simulink model "dynamicANN"  (R2019b)
settings: Solver=VariableStepAuto  StartTime=0.0  StopTime=3  RelTol=1e-3
values from neighbouring files (symbols this model uses):
  a = 87.548e-3    (= 0.087548)    [main.m]
  b = 132.452e-3    (= 0.132452)    [main.m]
  d = 22.452e-3    (= 0.022452)    [main.m]
  delta = 4e-6    (= 4e-06)    [main.m]
  F1 = mass*g-F2    (= 23.4474357109)    [main.m]
  F2 = a*mass*g/(a+b)    (= 15.4982642891)    [main.m]
  g = 9.81    [main.m]
  h0 = 75e-6    (= 7.5e-05)    [main.m]
  Jd = 0.047331604    [main.m]
  Jp = 0.00075    [main.m]
  Kps = (Vmax-Vmin)/(Hmax-Hmin)    (= 1666.66666667)    [main.m]
  Ksv = 30    [main.m]
  mass = 3.970    (= 3.97)    [main.m]
  mm = F2/g    (= 1.57984345455)    [main.m]
  omega = n_rpm*2*pi/60    (= 293.215314335)    [main.m]
  s = 30e-3    (= 0.03)    [main.m]
  tau = 0.12    [main.m]
  taus = 0.00125    [main.m]
  Ts = 1/fs    (= 0.001)    [main.m]
libraries: neural x480, simulink x2
(part 4 of 11)

== system dynamicANN/BEARING 1 NL1/B1NN/Layer 2/Delays 1 ==
  "p{2}" : Inport  PortDimensions=100
      mask Display: e = 0.06;c1 = [120 230 180]/255;c2 = ([120 230 180]+0)/(256+128);c3 = ([120 230 180]+128)/(256+128);patch([0 1 1 0],[0 0 1 1],c1);patch([0 1 1 1-e 1-e 0+e],[0 0 1 1-e 0+e 0+e],c2);patch([0 0 1 1-e 0+e 0+e],[0 1 1 1-e 1-e 0+e],c3);plot([0 1 1 0 0],[0 0 1 1 0]);
  mux : Mux  Inputs=1
      mask Display: e = 0.06;c1 = [120 150 230]/255;c2 = ([120 150 230]+0)/383;c3 = ([120 150 230]+128)/383;patch([0 1 1 0],[0 0 1 1],c1);patch([0 1 1 1-e 1-e 0+e],[0 0 1 1-e 0+e 0+e],c2);patch([0 0 1 1-e 0+e 0+e],[0 1 1 1-e 1-e 0+e],c3);plot([0 1 1 0 0],[0 0 1 1 0]);disp('Mux')
  "pd{2,1}" : Outport
      mask Display: e = 0.06;c1 = [120 230 180]/255;c2 = ([120 230 180]+0)/(256+128);c3 = ([120 230 180]+128)/(256+128);patch([0 1 1 0],[0 0 1 1],c1);patch([0 1 1 1-e 1-e 0+e],[0 0 1 1-e 0+e 0+e],c2);patch([0 0 1 1-e 0+e 0+e],[0 1 1 1-e 1-e 0+e],c3);plot([0 1 1 0 0],[0 0 1 1 0]);
  wires:
  "p{2}"/1 -> mux/1
  mux/1 -> "pd{2,1}"/1

== system dynamicANN/BEARING 1 NL1/B1NN/Layer 2/LW{2,1} ==
  "ad{2,1}" : Inport  PortDimensions=100
      mask Display: e = 0.06;c1 = [120 230 180]/255;c2 = ([120 230 180]+0)/(256+128);c3 = ([120 230 180]+128)/(256+128);patch([0 1 1 0],[0 0 1 1],c1);patch([0 1 1 1-e 1-e 0+e],[0 0 1 1-e 0+e 0+e],c2);patch([0 0 1 1-e 0+e 0+e],[0 1 1 1-e 1-e 0+e],c3);plot([0 1 1 0 0],[0 0 1 1 0]);
  "IW{2,1}(1,:)'" : Constant  Value=[0.1698079109499475991551520337452529929578304290771484375;0.290838474167385674373775827916688285768032073974609375;-2.22730984445659441206544215674512088298797607421875;-1.624079785730641045660149757168255746364593505859375;0.7981202553212247696734493729309178888797760009765625;-0.90370496781212639181291024215170182287693023681640625;1.2464100435990104198680228364537470042705535888671875;1.63415315773707536806114148930646479129791259765625;-0.810684982726251224249836013768799602985382080078125;2.493795827263717956867594693903811275959014892578125;-0.97637144815646281781340576344518922269344329833984375;-0.61194362554906411855171199931646697223186492919921875;-0.69885511961833002292365790708572603762149810791015625;-0.1345882708286832707411662113372585736215114593505859375;0.76822779076666536379747185492306016385555267333984375;-0.307473182269908329455887496806099079549312591552734375;-0.56982199636107611073754242170252837240695953369140625;4.39259906999470484123548885690979659557342529296875;-0.06382692473601613014633215925641707144677639007568359375;-0.7337819449502240853888679339434020221233367919921875;-0.74015310276954948687233581949840299785137176513671875;1.4095461284749808417160465978668071329593658447265625;1.5372200397936139903976027198950760066509246826171875;-0.70566939576721809945780705675133503973484039306640625;-1.4184873848022065967455773716210387647151947021484375;0.86210795579773991104133301632828079164028167724609375;-1.8451474979371036422293173018260858952999114990234375;0.8609497543302595534697729817708022892475128173828125;1.65789076993955131200664254720322787761688232421875;-1.1369511449201945563203253186657093465328216552734375;-0.62812441329608947881979474914260208606719970703125;1.742409455756594116593305443529970943927764892578125;0.75348495824883487959056083127507008612155914306640625;-0.982876727594547361377408378757536411285400390625;0.271928521471438255918684490097803063690662384033203125;-0.413283020475831819329215477409888990223407745361328125;0.360701116369382790427522422760375775396823883056640625;-0.65188523559179412103503636899404227733612060546875;0.805574788685706533186703381943516433238983154296875;2.8430251715888683605726328096352517604827880859375;-0.28892335685882042373151534775388427078723907470703125;-0.91624640165756499055049744129064492881298065185546875;2.11165661214157562852733462932519614696502685546875;-3.384488322878890453893063750001601874828338623046875;2.61269214159002860498048903536982834339141845703125;2.01213120374260068246030641603283584117889404296875;-1.846846419579796449994546492234803736209869384765625;-0.1927495993139352881140524686998105607926845550537109375;0.322981729667515982118430883929249830543994903564453125;-0.73499935329750509804824787352117709815502166748046875;6.8127582971923192900476351496763527393341064453125;0.6096740827140967322606002198881469666957855224609375;-1.846639270374431429644346280838362872600555419921875;-0.86829506880616325048549697385169565677642822265625;1.5492791813355781815886302865692414343357086181640625;0.0945451987484815237205992843882995657622814178466796875;1.0488742019501973157247221024590544402599334716796875;-2.184927166768952933040282005094923079013824462890625;-0.0858346683681262823117918969728634692728519439697265625;0.76949205911817042391476206830702722072601318359375;-1.0985151425390622392797013162635266780853271484375;-2.543759677786384454378776354133151471614837646484375;-0.470946206200558215027029973498429171741008758544921875;-1.53318014231124433166542075923644006252288818359375;1.061736469851976227829482013476081192493438720703125;1.5135219730075204491726026390097104012966156005859375;0.3122388005480136730085405361023731529712677001953125;-1.106440417092606320892400617594830691814422607421875;-0.11002187691186014750766020142691559158265590667724609375;1.5886326101169714331007298824260942637920379638671875;2.1009464962127264442415253142826259136199951171875;0.4290224342034452131855459811049513518810272216796875 ...(+1546 chars)]
      mask Display: e = 0.06;c1 = [120 150 230]/255;c2 = ([120 150 230]+0)/383;c3 = ([120 150 230]+128)/383;patch([0 1 1 0],[0 0 1 1],c1);patch([0 1 1 1-e 1-e 0+e],[0 0 1 1-e 0+e 0+e],c2);patch([0 0 1 1-e 0+e 0+e],[0 1 1 1-e 1-e 0+e],c3);plot([0 1 1 0 0],[0 0 1 1 0]);disp('weights');
  "IW{2,1}(2,:)'" : Constant  Value=[-0.376849018375156219473609553460846655070781707763671875;2.53110949685541886111650455859489738941192626953125;0.11614639993883658919404666676200577057898044586181640625;-0.17028397802693862050915640793391503393650054931640625;0.300872698834586282945480206763022579252719879150390625;-0.84058409961180979852457539891474880278110504150390625;-0.8337115620731412324317943784990347921848297119140625;-0.5963344064050686288425140446634031832218170166015625;0.10360853973076906975325783832886372692883014678955078125;-0.188200258423388111506113773430115543305873870849609375;0.371617718509079930644389833105378784239292144775390625;-0.60717811263409415811764802128891460597515106201171875;3.360163111521968115624758866033516824245452880859375;2.388875554686178848129429752589203417301177978515625;-0.80876161108209709826866173898451961576938629150390625;0.40698967487644888141318233465426601469516754150390625;0.3087777698698708217506236906046979129314422607421875;0.452639706492497018164300470743910409510135650634765625;-1.415289712366708752000477034016512334346771240234375;1.11519101040323764806316830799914896488189697265625;-0.74108359067836471201218273563426919281482696533203125;-4.38392461551207102132821091799996793270111083984375;-1.1748164412167876324843973634415306150913238525390625;-4.59326123502451455493655885220505297183990478515625;0.68020562799390138497557245500502176582813262939453125;-0.9090416930932245787033707529189996421337127685546875;-1.22682373665466482037800233229063451290130615234375;-1.7497069826856399554770860049757175147533416748046875;1.4849313464642026616502334945835173130035400390625;-0.36809309421732050449094231225899420678615570068359375;-0.72048459319552027313449116263655014336109161376953125;-0.447880935563048920844408939956338144838809967041015625;1.2235940470277257841047457986860536038875579833984375;-3.2335347484420129404725230415351688861846923828125;1.979918112877920410852539134793914854526519775390625;-4.92410310158344000086572123109363019466400146484375;-2.093909056470530938298679757281206548213958740234375;0.64465935007834185288544404102140106260776519775390625;-0.343533958918883886024531193470465950667858123779296875;-0.97616487204412349942828086568624712526798248291015625;2.173662143267287572001578155322931706905364990234375;3.075972814595175020002670862595550715923309326171875;0.005623696695469050481352990544792191940359771251678466796875;2.52820578269359241829761231201700866222381591796875;1.39894121160601248021748688188381493091583251953125;0.7848170956726494562616380790132097899913787841796875;0.28850790735402076503390844663954339921474456787109375;-1.4589627667777589348219180465093813836574554443359375;-0.050217068099909077660836231871144264005124568939208984375;0.250564798154844503574878444851492531597614288330078125;-0.4099543262265734622218360527767799794673919677734375;0.669301069966697692592560997582040727138519287109375;-1.026297510686760450226984175969846546649932861328125;-0.37085687778584974783058214597986079752445220947265625;0.994229602951526292287098840461112558841705322265625;-0.04131868769835296550940739734869566746056079864501953125;-2.390357445245252510090949726873077452182769775390625;-0.77468288425896825177829896347247995436191558837890625;-1.893031061665151337791712649050168693065643310546875;5.46564472431920034267704977537505328655242919921875;0.6814522142056798070797185573610477149486541748046875;-6.9524690097170047664576486567966639995574951171875;-0.70352271530726195880589557418716140091419219970703125;0.64012929736886281517627139692194759845733642578125;-0.68910894849149684215916522589395754039287567138671875;1.555987744074827094920010495116002857685089111328125;0.5092286159042431759047531159012578427791595458984375;-1.69190110493891854304138178122229874134063720703125;-0.391682270640478502610193345390143804252147674560546875;-0.0189285477103646980479023653742842725478112697601318359375;1.8648133866790299606464031967334449291229248046875 ...(+1619 chars)]
      mask Display: e = 0.06;c1 = [120 150 230]/255;c2 = ([120 150 230]+0)/383;c3 = ([120 150 230]+128)/383;patch([0 1 1 0],[0 0 1 1],c1);patch([0 1 1 1-e 1-e 0+e],[0 0 1 1-e 0+e 0+e],c2);patch([0 0 1 1-e 0+e 0+e],[0 1 1 1-e 1-e 0+e],c3);plot([0 1 1 0 0],[0 0 1 1 0]);disp('weights');
  Mux : Mux  Inputs=2
      mask Display: e = 0.06;c1 = [120 150 230]/255;c2 = ([120 150 230]+0)/383;c3 = ([120 150 230]+128)/383;patch([0 1 1 0],[0 0 1 1],c1);patch([0 1 1 1-e 1-e 0+e],[0 0 1 1-e 0+e 0+e],c2);patch([0 0 1 1-e 0+e 0+e],[0 1 1 1-e 1-e 0+e],c3);plot([0 1 1 0 0],[0 0 1 1 0]);disp('Mux');
  dotprod1 : neural/Weight Functions/dotprod
      settings: SourceProductName=Deep Learning Toolbox
  dotprod2 : neural/Weight Functions/dotprod
      settings: SourceProductName=Deep Learning Toolbox
  "lz{2,1}" : Outport
      mask Display: e = 0.06;c1 = [120 230 180]/255;c2 = ([120 230 180]+0)/(256+128);c3 = ([120 230 180]+128)/(256+128);patch([0 1 1 0],[0 0 1 1],c1);patch([0 1 1 1-e 1-e 0+e],[0 0 1 1-e 0+e 0+e],c2);patch([0 0 1 1-e 0+e 0+e],[0 1 1 1-e 1-e 0+e],c3);plot([0 1 1 0 0],[0 0 1 1 0]);
  wires:
  "IW{2,1}(1,:)'"/1 -> dotprod1/1
  "ad{2,1}"/1 -> dotprod1/2, dotprod2/2
  dotprod1/1 -> Mux/1
  "IW{2,1}(2,:)'"/1 -> dotprod2/1
  dotprod2/1 -> Mux/2
  Mux/1 -> "lz{2,1}"/1

== system dynamicANN/BEARING 2 NL1/B2NN /Layer 1/Delays 1 ==
  "p{1}" : Inport  PortDimensions=4
      mask Display: e = 0.06;c1 = [120 230 180]/255;c2 = ([120 230 180]+0)/(256+128);c3 = ([120 230 180]+128)/(256+128);patch([0 1 1 0],[0 0 1 1],c1);patch([0 1 1 1-e 1-e 0+e],[0 0 1 1-e 0+e 0+e],c2);patch([0 0 1 1-e 0+e 0+e],[0 1 1 1-e 1-e 0+e],c3);plot([0 1 1 0 0],[0 0 1 1 0]);
  mux : Mux  Inputs=1
      mask Display: e = 0.06;c1 = [120 150 230]/255;c2 = ([120 150 230]+0)/383;c3 = ([120 150 230]+128)/383;patch([0 1 1 0],[0 0 1 1],c1);patch([0 1 1 1-e 1-e 0+e],[0 0 1 1-e 0+e 0+e],c2);patch([0 0 1 1-e 0+e 0+e],[0 1 1 1-e 1-e 0+e],c3);plot([0 1 1 0 0],[0 0 1 1 0]);disp('Mux')
  "pd{1,1}" : Outport
      mask Display: e = 0.06;c1 = [120 230 180]/255;c2 = ([120 230 180]+0)/(256+128);c3 = ([120 230 180]+128)/(256+128);patch([0 1 1 0],[0 0 1 1],c1);patch([0 1 1 1-e 1-e 0+e],[0 0 1 1-e 0+e 0+e],c2);patch([0 0 1 1-e 0+e 0+e],[0 1 1 1-e 1-e 0+e],c3);plot([0 1 1 0 0],[0 0 1 1 0]);
  wires:
  "p{1}"/1 -> mux/1
  mux/1 -> "pd{1,1}"/1
